simulink model "gm_DSBF"  (R2019b)
settings: Solver=FixedStepDiscrete  StartTime=0.0  StopTime=0.02  RelTol=1e-3
InitFcn:
  | sm_callback_init
StopFcn:
  | sm_callback_stop
undefined symbols (not defined in the file or in its folder): arraySize, arraySpacing, delayDataTypeFractionLength, delayDataTypeSign, delayDataTypeWordLength, mp, samplingRate, speedOfSound, upsampleFactor
libraries: hdlsllib x64, simulink x36, dspmlti4 x16, dsphdlfiltering x16
(part 3 of 5)

== system gm_DSBF/dataplane/Avalon Data Processing/delay signals_instance4/delay signal ==
  note: CIC interpolation
  note: Integer delay
  note: fractional delay (upsampled)
  data_in : Inport  OutDataTypeStr=fixdt(1, 32, 28)  PortDimensions=1  SampleTime=2.08333333333333e-05
  delay : Inport  Port=2  OutDataTypeStr=fixdt(1, 12, 6)  PortDimensions=1  SampleTime=2.08333333333333e-05
  CIC Interpolation : dspmlti4/CIC Interpolation  filtFrom=Filter object  filtobj=mp.cicInterpolator  ftype=Interpolator  R=mp.upsampleFactor  M=1  N=2  filterInternals=Full precision  BPS=[16 16 16 16]  FLPS=0  outputWordLength=32  outputFracLength=0  launchFVT=off  framing=Allow multirate processing  OutputFrames=off
      settings: SourceProductName=DSP System Toolbox  SourceProductBaseCode=DS
  CIC interpolation compensator : dsphdlfiltering/Discrete FIR Filter HDL Optimized  NumeratorSource=Property  Numerator=mp.cicInterpolatorCompensator.coeffs.Numerator  NumeratorPrototype=[]  FilterStructure=Direct form systolic  SerializationOption=Maximum number of multipliers  NumberOfCycles=2  NumberOfMultipliers=4  SimulateUsing=Code generation  roundingMode=Floor  overflowMode=off  CoefficientsDataTypeStr=fixdt(1,16)  CoefficientsMin=[]  CoefficientsMax=[]  OutputDataTypeStr=Inherit: Same word length as input  OutputMin=[]  OutputMax=[]  ResetInputPort=off  HDLGlobalReset=off
      settings: SourceProductName=DSP System Toolbox  SourceProductBaseCode=DS
  CIC interpolation gain compensation : ArithShift  BitShiftNumber=4  BinPtShiftNumber=double(0)
  Constant : Constant  OutDataTypeStr=boolean  SampleTime=-1
  Constant1 : Constant  OutDataTypeStr=boolean  SampleTime=-1
  Constant2 : Constant  OutDataTypeStr=boolean  SampleTime=-1
  Data Type Conversion : DataTypeConversion  OutDataTypeStr=fixdt(1, 32, 28)  SampleTime=1.30208333333333e-06
  Data Type Conversion1 : DataTypeConversion  OutDataTypeStr=fixdt(1, 32, 28)  SampleTime=2.08333333333333e-05
  Downsample : DownSample  N=double(16)  phase=double(0)  RateOptions=Allow multirate processing
  PipelineRegister : Delay  DelayLength=double(1)  InitialCondition=0  SampleTime=2.08333333333333e-05
  Rate Transition : RateTransition  InitialCondition=double(0)  OutPortSampleTimeOpt=Multiple of input port sample time  OutPortSampleTimeMultiple=1/16
  Rate Transition1 : RateTransition  InitialCondition=double(0)  OutPortSampleTimeOpt=Multiple of input port sample time  OutPortSampleTimeMultiple=1/2048
  Terminator2 : Terminator
  delayMatch{,1..3} (4 alike) : Delay  DelayLength=double(2)  InitialCondition=0  SampleTime=2.08333333333333e-05
  delayMatch4 : Delay  DelayLength=double(32)  InitialCondition=0  SampleTime=1.30208333333333e-06
  delayMatch5 : Delay  DelayLength=double(32)  InitialCondition=0  SampleTime=1.30208333333333e-06
  delayMatch6 : Delay  DelayLength=double(32)  InitialCondition=0  SampleTime=1.30208333333333e-06
  fractional delay DPRAM : hdlsllib/HDL RAMs/Simple Dual Port RAM  ram_size=mp.fractionalDelayAddrSize
      settings: SourceProductName=Simulink  SourceProductBaseCode=SL
  integer delay DPRAM : hdlsllib/HDL RAMs/Simple Dual Port RAM  ram_size=mp.integerDelayAddrSize
      settings: SourceProductName=Simulink  SourceProductBaseCode=SL
  read address generator : Subsystem
  read address generator1 : Subsystem
  split_into_int_and_frac_parts : Subsystem
  write address generator : hdlsllib/Sources/HDL Counter  CountType=Count limited  CountInit=double(0)  CountStep=double(1)  CountMax=double(63)  CountFromType=Initial value  CountFrom=double(0)  CountResetPort=off  CountLoadPort=off  CountEnbPort=off  CountDirPort=off  CountDataType=Unsigned  CountWordLen=6  CountFracLen=0  CountSampTime=2.08333333333333e-05
      settings: SourceProductName=Simulink
  write address generator1 : hdlsllib/Sources/HDL Counter  CountType=Count limited  CountInit=double(0)  CountStep=double(1)  CountMax=double(63)  CountFromType=Initial value  CountFrom=double(0)  CountResetPort=off  CountLoadPort=off  CountEnbPort=off  CountDirPort=off  CountDataType=Unsigned  CountWordLen=6  CountFracLen=0  CountSampTime=1.30208333333333e-06
      settings: SourceProductName=Simulink
  data_out : Outport  VectorParamsAs1DForOutWhenUnconnected=off
  wires:
  Downsample/1 -> PipelineRegister/1
  CIC interpolation gain compensation/1 -> Data Type Conversion/1
  split_into_int_and_frac_parts/1(integer_delay) -> read address generator/2(delay)
  Constant1/1 -> delayMatch6/1
  write address generator1/1 -> delayMatch4/1, delayMatch5/1
  delayMatch5/1 -> fractional delay DPRAM/2
  Constant/1 -> delayMatch3/1
  Constant2/1 -> delayMatch2/1
  write address generator/1 -> delayMatch/1, delayMatch1/1
  delayMatch1/1 -> integer delay DPRAM/2
  delay/1 -> split_into_int_and_frac_parts/1(delay)
  data_in/1 -> integer delay DPRAM/1
  delayMatch3/1 -> CIC interpolation compensator/2
  delayMatch6/1 -> fractional delay DPRAM/3
  delayMatch2/1 -> integer delay DPRAM/3
  Data Type Conversion/1 -> fractional delay DPRAM/1
  Data Type Conversion1/1 -> Rate Transition1/1
  split_into_int_and_frac_parts/2(fractional_delay) -> Rate Transition/1
  read address generator/1(read_addr) -> integer delay DPRAM/4
  read address generator1/1(read_addr) -> fractional delay DPRAM/4
  CIC Interpolation/1 -> CIC interpolation gain compensation/1
  CIC interpolation compensator/2 -> Terminator2/1
  CIC interpolation compensator/1 -> CIC Interpolation/1
  PipelineRegister/1 -> Data Type Conversion1/1
  Rate Transition/1 -> read address generator1/2(delay)
  Rate Transition1/1 -> data_out/1
  fractional delay DPRAM/1 -> Downsample/1
  integer delay DPRAM/1 -> CIC interpolation compensator/1
  delayMatch/1 -> read address generator/1(write_addr)
  delayMatch4/1 -> read address generator1/1(write_addr)

== system gm_DSBF/dataplane/Avalon Data Processing/delay signals_instance5/delay signal ==
  note: CIC interpolation
  note: Integer delay
  note: fractional delay (upsampled)
  data_in : Inport  OutDataTypeStr=fixdt(1, 32, 28)  PortDimensions=1  SampleTime=2.08333333333333e-05
  delay : Inport  Port=2  OutDataTypeStr=fixdt(1, 12, 6)  PortDimensions=1  SampleTime=2.08333333333333e-05
  CIC Interpolation : dspmlti4/CIC Interpolation  filtFrom=Filter object  filtobj=mp.cicInterpolator  ftype=Interpolator  R=mp.upsampleFactor  M=1  N=2  filterInternals=Full precision  BPS=[16 16 16 16]  FLPS=0  outputWordLength=32  outputFracLength=0  launchFVT=off  framing=Allow multirate processing  OutputFrames=off
      settings: SourceProductName=DSP System Toolbox  SourceProductBaseCode=DS
  CIC interpolation compensator : dsphdlfiltering/Discrete FIR Filter HDL Optimized  NumeratorSource=Property  Numerator=mp.cicInterpolatorCompensator.coeffs.Numerator  NumeratorPrototype=[]  FilterStructure=Direct form systolic  SerializationOption=Maximum number of multipliers  NumberOfCycles=2  NumberOfMultipliers=4  SimulateUsing=Code generation  roundingMode=Floor  overflowMode=off  CoefficientsDataTypeStr=fixdt(1,16)  CoefficientsMin=[]  CoefficientsMax=[]  OutputDataTypeStr=Inherit: Same word length as input  OutputMin=[]  OutputMax=[]  ResetInputPort=off  HDLGlobalReset=off
      settings: SourceProductName=DSP System Toolbox  SourceProductBaseCode=DS
  CIC interpolation gain compensation : ArithShift  BitShiftNumber=4  BinPtShiftNumber=double(0)
  Constant : Constant  OutDataTypeStr=boolean  SampleTime=-1
  Constant1 : Constant  OutDataTypeStr=boolean  SampleTime=-1
  Constant2 : Constant  OutDataTypeStr=boolean  SampleTime=-1
  Data Type Conversion : DataTypeConversion  OutDataTypeStr=fixdt(1, 32, 28)  SampleTime=1.30208333333333e-06
  Data Type Conversion1 : DataTypeConversion  OutDataTypeStr=fixdt(1, 32, 28)  SampleTime=2.08333333333333e-05
  Downsample : DownSample  N=double(16)  phase=double(0)  RateOptions=Allow multirate processing
  PipelineRegister : Delay  DelayLength=double(1)  InitialCondition=0  SampleTime=2.08333333333333e-05
  Rate Transition : RateTransition  InitialCondition=double(0)  OutPortSampleTimeOpt=Multiple of input port sample time  OutPortSampleTimeMultiple=1/16
  Rate Transition1 : RateTransition  InitialCondition=double(0)  OutPortSampleTimeOpt=Multiple of input port sample time  OutPortSampleTimeMultiple=1/2048
  Terminator2 : Terminator
  delayMatch{,1..3} (4 alike) : Delay  DelayLength=double(2)  InitialCondition=0  SampleTime=2.08333333333333e-05
  delayMatch4 : Delay  DelayLength=double(32)  InitialCondition=0  SampleTime=1.30208333333333e-06
  delayMatch5 : Delay  DelayLength=double(32)  InitialCondition=0  SampleTime=1.30208333333333e-06
  delayMatch6 : Delay  DelayLength=double(32)  InitialCondition=0  SampleTime=1.30208333333333e-06
  fractional delay DPRAM : hdlsllib/HDL RAMs/Simple Dual Port RAM  ram_size=mp.fractionalDelayAddrSize
      settings: SourceProductName=Simulink  SourceProductBaseCode=SL
  integer delay DPRAM : hdlsllib/HDL RAMs/Simple Dual Port RAM  ram_size=mp.integerDelayAddrSize
      settings: SourceProductName=Simulink  SourceProductBaseCode=SL
  read address generator : Subsystem
  read address generator1 : Subsystem
  split_into_int_and_frac_parts : Subsystem
  write address generator : hdlsllib/Sources/HDL Counter  CountType=Count limited  CountInit=double(0)  CountStep=double(1)  CountMax=double(63)  CountFromType=Initial value  CountFrom=double(0)  CountResetPort=off  CountLoadPort=off  CountEnbPort=off  CountDirPort=off  CountDataType=Unsigned  CountWordLen=6  CountFracLen=0  CountSampTime=2.08333333333333e-05
      settings: SourceProductName=Simulink
  write address generator1 : hdlsllib/Sources/HDL Counter  CountType=Count limited  CountInit=double(0)  CountStep=double(1)  CountMax=double(63)  CountFromType=Initial value  CountFrom=double(0)  CountResetPort=off  CountLoadPort=off  CountEnbPort=off  CountDirPort=off  CountDataType=Unsigned  CountWordLen=6  CountFracLen=0  CountSampTime=1.30208333333333e-06
      settings: SourceProductName=Simulink
  data_out : Outport  VectorParamsAs1DForOutWhenUnconnected=off
  wires:
  Downsample/1 -> PipelineRegister/1
  CIC interpolation gain compensation/1 -> Data Type Conversion/1
  split_into_int_and_frac_parts/1(integer_delay) -> read address generator/2(delay)
  Constant1/1 -> delayMatch6/1
  write address generator1/1 -> delayMatch4/1, delayMatch5/1
  delayMatch5/1 -> fractional delay DPRAM/2
  Constant/1 -> delayMatch3/1
  Constant2/1 -> delayMatch2/1
  write address generator/1 -> delayMatch/1, delayMatch1/1
  delayMatch1/1 -> integer delay DPRAM/2
  delay/1 -> split_into_int_and_frac_parts/1(delay)
  data_in/1 -> integer delay DPRAM/1
  delayMatch3/1 -> CIC interpolation compensator/2
  delayMatch6/1 -> fractional delay DPRAM/3
  delayMatch2/1 -> integer delay DPRAM/3
  Data Type Conversion/1 -> fractional delay DPRAM/1
  Data Type Conversion1/1 -> Rate Transition1/1
  split_into_int_and_frac_parts/2(fractional_delay) -> Rate Transition/1
  read address generator/1(read_addr) -> integer delay DPRAM/4
  read address generator1/1(read_addr) -> fractional delay DPRAM/4
  CIC Interpolation/1 -> CIC interpolation gain compensation/1
  CIC interpolation compensator/2 -> Terminator2/1
  CIC interpolation compensator/1 -> CIC Interpolation/1
  PipelineRegister/1 -> Data Type Conversion1/1
  Rate Transition/1 -> read address generator1/2(delay)
  Rate Transition1/1 -> data_out/1
  fractional delay DPRAM/1 -> Downsample/1
  integer delay DPRAM/1 -> CIC interpolation compensator/1
  delayMatch/1 -> read address generator/1(write_addr)
  delayMatch4/1 -> read address generator1/1(write_addr)

== system gm_DSBF/dataplane/Avalon Data Processing/delay signals_instance6/delay signal ==
  note: CIC interpolation
  note: Integer delay
  note: fractional delay (upsampled)
  data_in : Inport  OutDataTypeStr=fixdt(1, 32, 28)  PortDimensions=1  SampleTime=2.08333333333333e-05
  delay : Inport  Port=2  OutDataTypeStr=fixdt(1, 12, 6)  PortDimensions=1  SampleTime=2.08333333333333e-05
  CIC Interpolation : dspmlti4/CIC Interpolation  filtFrom=Filter object  filtobj=mp.cicInterpolator  ftype=Interpolator  R=mp.upsampleFactor  M=1  N=2  filterInternals=Full precision  BPS=[16 16 16 16]  FLPS=0  outputWordLength=32  outputFracLength=0  launchFVT=off  framing=Allow multirate processing  OutputFrames=off
      settings: SourceProductName=DSP System Toolbox  SourceProductBaseCode=DS
  CIC interpolation compensator : dsphdlfiltering/Discrete FIR Filter HDL Optimized  NumeratorSource=Property  Numerator=mp.cicInterpolatorCompensator.coeffs.Numerator  NumeratorPrototype=[]  FilterStructure=Direct form systolic  SerializationOption=Maximum number of multipliers  NumberOfCycles=2  NumberOfMultipliers=4  SimulateUsing=Code generation  roundingMode=Floor  overflowMode=off  CoefficientsDataTypeStr=fixdt(1,16)  CoefficientsMin=[]  CoefficientsMax=[]  OutputDataTypeStr=Inherit: Same word length as input  OutputMin=[]  OutputMax=[]  ResetInputPort=off  HDLGlobalReset=off
      settings: SourceProductName=DSP System Toolbox  SourceProductBaseCode=DS
  CIC interpolation gain compensation : ArithShift  BitShiftNumber=4  BinPtShiftNumber=double(0)
  Constant : Constant  OutDataTypeStr=boolean  SampleTime=-1
  Constant1 : Constant  OutDataTypeStr=boolean  SampleTime=-1
  Constant2 : Constant  OutDataTypeStr=boolean  SampleTime=-1
  Data Type Conversion : DataTypeConversion  OutDataTypeStr=fixdt(1, 32, 28)  SampleTime=1.30208333333333e-06
  Data Type Conversion1 : DataTypeConversion  OutDataTypeStr=fixdt(1, 32, 28)  SampleTime=2.08333333333333e-05
  Downsample : DownSample  N=double(16)  phase=double(0)  RateOptions=Allow multirate processing
  PipelineRegister : Delay  DelayLength=double(1)  InitialCondition=0  SampleTime=2.08333333333333e-05
  Rate Transition : RateTransition  InitialCondition=double(0)  OutPortSampleTimeOpt=Multiple of input port sample time  OutPortSampleTimeMultiple=1/16
  Rate Transition1 : RateTransition  InitialCondition=double(0)  OutPortSampleTimeOpt=Multiple of input port sample time  OutPortSampleTimeMultiple=1/2048
  Terminator2 : Terminator
  delayMatch{,1..3} (4 alike) : Delay  DelayLength=double(2)  InitialCondition=0  SampleTime=2.08333333333333e-05
  delayMatch4 : Delay  DelayLength=double(32)  InitialCondition=0  SampleTime=1.30208333333333e-06
  delayMatch5 : Delay  DelayLength=double(32)  InitialCondition=0  SampleTime=1.30208333333333e-06
  delayMatch6 : Delay  DelayLength=double(32)  InitialCondition=0  SampleTime=1.30208333333333e-06
  fractional delay DPRAM : hdlsllib/HDL RAMs/Simple Dual Port RAM  ram_size=mp.fractionalDelayAddrSize
      settings: SourceProductName=Simulink  SourceProductBaseCode=SL
  integer delay DPRAM : hdlsllib/HDL RAMs/Simple Dual Port RAM  ram_size=mp.integerDelayAddrSize
      settings: SourceProductName=Simulink  SourceProductBaseCode=SL
  read address generator : Subsystem
  read address generator1 : Subsystem
  split_into_int_and_frac_parts : Subsystem
  write address generator : hdlsllib/Sources/HDL Counter  CountType=Count limited  CountInit=double(0)  CountStep=double(1)  CountMax=double(63)  CountFromType=Initial value  CountFrom=double(0)  CountResetPort=off  CountLoadPort=off  CountEnbPort=off  CountDirPort=off  CountDataType=Unsigned  CountWordLen=6  CountFracLen=0  CountSampTime=2.08333333333333e-05
      settings: SourceProductName=Simulink
  write address generator1 : hdlsllib/Sources/HDL Counter  CountType=Count limited  CountInit=double(0)  CountStep=double(1)  CountMax=double(63)  CountFromType=Initial value  CountFrom=double(0)  CountResetPort=off  CountLoadPort=off  CountEnbPort=off  CountDirPort=off  CountDataType=Unsigned  CountWordLen=6  CountFracLen=0  CountSampTime=1.30208333333333e-06
      settings: SourceProductName=Simulink
  data_out : Outport  VectorParamsAs1DForOutWhenUnconnected=off
  wires:
  Downsample/1 -> PipelineRegister/1
  CIC interpolation gain compensation/1 -> Data Type Conversion/1
  split_into_int_and_frac_parts/1(integer_delay) -> read address generator/2(delay)
  Constant1/1 -> delayMatch6/1
  write address generator1/1 -> delayMatch4/1, delayMatch5/1
  delayMatch5/1 -> fractional delay DPRAM/2
  Constant/1 -> delayMatch3/1
  Constant2/1 -> delayMatch2/1
  write address generator/1 -> delayMatch/1, delayMatch1/1
  delayMatch1/1 -> integer delay DPRAM/2
  delay/1 -> split_into_int_and_frac_parts/1(delay)
  data_in/1 -> integer delay DPRAM/1
  delayMatch3/1 -> CIC interpolation compensator/2
  delayMatch6/1 -> fractional delay DPRAM/3
  delayMatch2/1 -> integer delay DPRAM/3
  Data Type Conversion/1 -> fractional delay DPRAM/1
  Data Type Conversion1/1 -> Rate Transition1/1
  split_into_int_and_frac_parts/2(fractional_delay) -> Rate Transition/1
  read address generator/1(read_addr) -> integer delay DPRAM/4
  read address generator1/1(read_addr) -> fractional delay DPRAM/4
  CIC Interpolation/1 -> CIC interpolation gain compensation/1
  CIC interpolation compensator/2 -> Terminator2/1
  CIC interpolation compensator/1 -> CIC Interpolation/1
  PipelineRegister/1 -> Data Type Conversion1/1
  Rate Transition/1 -> read address generator1/2(delay)
  Rate Transition1/1 -> data_out/1
  fractional delay DPRAM/1 -> Downsample/1
  integer delay DPRAM/1 -> CIC interpolation compensator/1
  delayMatch/1 -> read address generator/1(write_addr)
  delayMatch4/1 -> read address generator1/1(write_addr)

== system gm_DSBF/dataplane/Avalon Data Processing/delay signals_instance7/delay signal ==
  note: CIC interpolation
  note: Integer delay
  note: fractional delay (upsampled)
  data_in : Inport  OutDataTypeStr=fixdt(1, 32, 28)  PortDimensions=1  SampleTime=2.08333333333333e-05
  delay : Inport  Port=2  OutDataTypeStr=fixdt(1, 12, 6)  PortDimensions=1  SampleTime=2.08333333333333e-05
  CIC Interpolation : dspmlti4/CIC Interpolation  filtFrom=Filter object  filtobj=mp.cicInterpolator  ftype=Interpolator  R=mp.upsampleFactor  M=1  N=2  filterInternals=Full precision  BPS=[16 16 16 16]  FLPS=0  outputWordLength=32  outputFracLength=0  launchFVT=off  framing=Allow multirate processing  OutputFrames=off
      settings: SourceProductName=DSP System Toolbox  SourceProductBaseCode=DS
  CIC interpolation compensator : dsphdlfiltering/Discrete FIR Filter HDL Optimized  NumeratorSource=Property  Numerator=mp.cicInterpolatorCompensator.coeffs.Numerator  NumeratorPrototype=[]  FilterStructure=Direct form systolic  SerializationOption=Maximum number of multipliers  NumberOfCycles=2  NumberOfMultipliers=4  SimulateUsing=Code generation  roundingMode=Floor  overflowMode=off  CoefficientsDataTypeStr=fixdt(1,16)  CoefficientsMin=[]  CoefficientsMax=[]  OutputDataTypeStr=Inherit: Same word length as input  OutputMin=[]  OutputMax=[]  ResetInputPort=off  HDLGlobalReset=off
      settings: SourceProductName=DSP System Toolbox  SourceProductBaseCode=DS
  CIC interpolation gain compensation : ArithShift  BitShiftNumber=4  BinPtShiftNumber=double(0)
  Constant : Constant  OutDataTypeStr=boolean  SampleTime=-1
  Constant1 : Constant  OutDataTypeStr=boolean  SampleTime=-1
  Constant2 : Constant  OutDataTypeStr=boolean  SampleTime=-1
  Data Type Conversion : DataTypeConversion  OutDataTypeStr=fixdt(1, 32, 28)  SampleTime=1.30208333333333e-06
  Data Type Conversion1 : DataTypeConversion  OutDataTypeStr=fixdt(1, 32, 28)  SampleTime=2.08333333333333e-05
  Downsample : DownSample  N=double(16)  phase=double(0)  RateOptions=Allow multirate processing
  PipelineRegister : Delay  DelayLength=double(1)  InitialCondition=0  SampleTime=2.08333333333333e-05
  Rate Transition : RateTransition  InitialCondition=double(0)  OutPortSampleTimeOpt=Multiple of input port sample time  OutPortSampleTimeMultiple=1/16
  Rate Transition1 : RateTransition  InitialCondition=double(0)  OutPortSampleTimeOpt=Multiple of input port sample time  OutPortSampleTimeMultiple=1/2048
  Terminator2 : Terminator
  delayMatch{,1..3} (4 alike) : Delay  DelayLength=double(2)  InitialCondition=0  SampleTime=2.08333333333333e-05
  delayMatch4 : Delay  DelayLength=double(32)  InitialCondition=0  SampleTime=1.30208333333333e-06
  delayMatch5 : Delay  DelayLength=double(32)  InitialCondition=0  SampleTime=1.30208333333333e-06
  delayMatch6 : Delay  DelayLength=double(32)  InitialCondition=0  SampleTime=1.30208333333333e-06
  fractional delay DPRAM : hdlsllib/HDL RAMs/Simple Dual Port RAM  ram_size=mp.fractionalDelayAddrSize
      settings: SourceProductName=Simulink  SourceProductBaseCode=SL
  integer delay DPRAM : hdlsllib/HDL RAMs/Simple Dual Port RAM  ram_size=mp.integerDelayAddrSize
      settings: SourceProductName=Simulink  SourceProductBaseCode=SL
  read address generator : Subsystem
  read address generator1 : Subsystem
  split_into_int_and_frac_parts : Subsystem
  write address generator : hdlsllib/Sources/HDL Counter  CountType=Count limited  CountInit=double(0)  CountStep=double(1)  CountMax=double(63)  CountFromType=Initial value  CountFrom=double(0)  CountResetPort=off  CountLoadPort=off  CountEnbPort=off  CountDirPort=off  CountDataType=Unsigned  CountWordLen=6  CountFracLen=0  CountSampTime=2.08333333333333e-05
      settings: SourceProductName=Simulink
  write address generator1 : hdlsllib/Sources/HDL Counter  CountType=Count limited  CountInit=double(0)  CountStep=double(1)  CountMax=double(63)  CountFromType=Initial value  CountFrom=double(0)  CountResetPort=off  CountLoadPort=off  CountEnbPort=off  CountDirPort=off  CountDataType=Unsigned  CountWordLen=6  CountFracLen=0  CountSampTime=1.30208333333333e-06
      settings: SourceProductName=Simulink
  data_out : Outport  VectorParamsAs1DForOutWhenUnconnected=off
  wires:
  Downsample/1 -> PipelineRegister/1
  CIC interpolation gain compensation/1 -> Data Type Conversion/1
  split_into_int_and_frac_parts/1(integer_delay) -> read address generator/2(delay)
  Constant1/1 -> delayMatch6/1
  write address generator1/1 -> delayMatch4/1, delayMatch5/1
  delayMatch5/1 -> fractional delay DPRAM/2
  Constant/1 -> delayMatch3/1
  Constant2/1 -> delayMatch2/1
  write address generator/1 -> delayMatch/1, delayMatch1/1
  delayMatch1/1 -> integer delay DPRAM/2
  delay/1 -> split_into_int_and_frac_parts/1(delay)
  data_in/1 -> integer delay DPRAM/1
  delayMatch3/1 -> CIC interpolation compensator/2
  delayMatch6/1 -> fractional delay DPRAM/3
  delayMatch2/1 -> integer delay DPRAM/3
  Data Type Conversion/1 -> fractional delay DPRAM/1
  Data Type Conversion1/1 -> Rate Transition1/1
  split_into_int_and_frac_parts/2(fractional_delay) -> Rate Transition/1
  read address generator/1(read_addr) -> integer delay DPRAM/4
  read address generator1/1(read_addr) -> fractional delay DPRAM/4
  CIC Interpolation/1 -> CIC interpolation gain compensation/1
  CIC interpolation compensator/2 -> Terminator2/1
  CIC interpolation compensator/1 -> CIC Interpolation/1
  PipelineRegister/1 -> Data Type Conversion1/1
  Rate Transition/1 -> read address generator1/2(delay)
  Rate Transition1/1 -> data_out/1
  fractional delay DPRAM/1 -> Downsample/1
  integer delay DPRAM/1 -> CIC interpolation compensator/1
  delayMatch/1 -> read address generator/1(write_addr)
  delayMatch4/1 -> read address generator1/1(write_addr)

== system gm_DSBF/dataplane/Avalon Data Processing/delay signals_instance8/delay signal ==
  note: CIC interpolation
  note: Integer delay
  note: fractional delay (upsampled)
  data_in : Inport  OutDataTypeStr=fixdt(1, 32, 28)  PortDimensions=1  SampleTime=2.08333333333333e-05
  delay : Inport  Port=2  OutDataTypeStr=fixdt(1, 12, 6)  PortDimensions=1  SampleTime=2.08333333333333e-05
  CIC Interpolation : dspmlti4/CIC Interpolation  filtFrom=Filter object  filtobj=mp.cicInterpolator  ftype=Interpolator  R=mp.upsampleFactor  M=1  N=2  filterInternals=Full precision  BPS=[16 16 16 16]  FLPS=0  outputWordLength=32  outputFracLength=0  launchFVT=off  framing=Allow multirate processing  OutputFrames=off
      settings: SourceProductName=DSP System Toolbox  SourceProductBaseCode=DS
  CIC interpolation compensator : dsphdlfiltering/Discrete FIR Filter HDL Optimized  NumeratorSource=Property  Numerator=mp.cicInterpolatorCompensator.coeffs.Numerator  NumeratorPrototype=[]  FilterStructure=Direct form systolic  SerializationOption=Maximum number of multipliers  NumberOfCycles=2  NumberOfMultipliers=4  SimulateUsing=Code generation  roundingMode=Floor  overflowMode=off  CoefficientsDataTypeStr=fixdt(1,16)  CoefficientsMin=[]  CoefficientsMax=[]  OutputDataTypeStr=Inherit: Same word length as input  OutputMin=[]  OutputMax=[]  ResetInputPort=off  HDLGlobalReset=off
      settings: SourceProductName=DSP System Toolbox  SourceProductBaseCode=DS
  CIC interpolation gain compensation : ArithShift  BitShiftNumber=4  BinPtShiftNumber=double(0)
  Constant : Constant  OutDataTypeStr=boolean  SampleTime=-1
  Constant1 : Constant  OutDataTypeStr=boolean  SampleTime=-1
  Constant2 : Constant  OutDataTypeStr=boolean  SampleTime=-1
  Data Type Conversion : DataTypeConversion  OutDataTypeStr=fixdt(1, 32, 28)  SampleTime=1.30208333333333e-06
  Data Type Conversion1 : DataTypeConversion  OutDataTypeStr=fixdt(1, 32, 28)  SampleTime=2.08333333333333e-05
  Downsample : DownSample  N=double(16)  phase=double(0)  RateOptions=Allow multirate processing
  PipelineRegister : Delay  DelayLength=double(1)  InitialCondition=0  SampleTime=2.08333333333333e-05
  Rate Transition : RateTransition  InitialCondition=double(0)  OutPortSampleTimeOpt=Multiple of input port sample time  OutPortSampleTimeMultiple=1/16
  Rate Transition1 : RateTransition  InitialCondition=double(0)  OutPortSampleTimeOpt=Multiple of input port sample time  OutPortSampleTimeMultiple=1/2048
  Terminator2 : Terminator
  delayMatch{,1..3} (4 alike) : Delay  DelayLength=double(2)  InitialCondition=0  SampleTime=2.08333333333333e-05
  delayMatch4 : Delay  DelayLength=double(32)  InitialCondition=0  SampleTime=1.30208333333333e-06
  delayMatch5 : Delay  DelayLength=double(32)  InitialCondition=0  SampleTime=1.30208333333333e-06
  delayMatch6 : Delay  DelayLength=double(32)  InitialCondition=0  SampleTime=1.30208333333333e-06
  fractional delay DPRAM : hdlsllib/HDL RAMs/Simple Dual Port RAM  ram_size=mp.fractionalDelayAddrSize
      settings: SourceProductName=Simulink  SourceProductBaseCode=SL
  integer delay DPRAM : hdlsllib/HDL RAMs/Simple Dual Port RAM  ram_size=mp.integerDelayAddrSize
      settings: SourceProductName=Simulink  SourceProductBaseCode=SL
  read address generator : Subsystem
  read address generator1 : Subsystem
  split_into_int_and_frac_parts : Subsystem
  write address generator : hdlsllib/Sources/HDL Counter  CountType=Count limited  CountInit=double(0)  CountStep=double(1)  CountMax=double(63)  CountFromType=Initial value  CountFrom=double(0)  CountResetPort=off  CountLoadPort=off  CountEnbPort=off  CountDirPort=off  CountDataType=Unsigned  CountWordLen=6  CountFracLen=0  CountSampTime=2.08333333333333e-05
      settings: SourceProductName=Simulink
  write address generator1 : hdlsllib/Sources/HDL Counter  CountType=Count limited  CountInit=double(0)  CountStep=double(1)  CountMax=double(63)  CountFromType=Initial value  CountFrom=double(0)  CountResetPort=off  CountLoadPort=off  CountEnbPort=off  CountDirPort=off  CountDataType=Unsigned  CountWordLen=6  CountFracLen=0  CountSampTime=1.30208333333333e-06
      settings: SourceProductName=Simulink
  data_out : Outport  VectorParamsAs1DForOutWhenUnconnected=off
  wires:
  Downsample/1 -> PipelineRegister/1
  CIC interpolation gain compensation/1 -> Data Type Conversion/1
  split_into_int_and_frac_parts/1(integer_delay) -> read address generator/2(delay)
  Constant1/1 -> delayMatch6/1
  write address generator1/1 -> delayMatch4/1, delayMatch5/1
  delayMatch5/1 -> fractional delay DPRAM/2
  Constant/1 -> delayMatch3/1
  Constant2/1 -> delayMatch2/1
  write address generator/1 -> delayMatch/1, delayMatch1/1
  delayMatch1/1 -> integer delay DPRAM/2
  delay/1 -> split_into_int_and_frac_parts/1(delay)
  data_in/1 -> integer delay DPRAM/1
  delayMatch3/1 -> CIC interpolation compensator/2
  delayMatch6/1 -> fractional delay DPRAM/3
  delayMatch2/1 -> integer delay DPRAM/3
  Data Type Conversion/1 -> fractional delay DPRAM/1
  Data Type Conversion1/1 -> Rate Transition1/1
  split_into_int_and_frac_parts/2(fractional_delay) -> Rate Transition/1
  read address generator/1(read_addr) -> integer delay DPRAM/4
  read address generator1/1(read_addr) -> fractional delay DPRAM/4
  CIC Interpolation/1 -> CIC interpolation gain compensation/1
  CIC interpolation compensator/2 -> Terminator2/1
  CIC interpolation compensator/1 -> CIC Interpolation/1
  PipelineRegister/1 -> Data Type Conversion1/1
  Rate Transition/1 -> read address generator1/2(delay)
  Rate Transition1/1 -> data_out/1
  fractional delay DPRAM/1 -> Downsample/1
  integer delay DPRAM/1 -> CIC interpolation compensator/1
  delayMatch/1 -> read address generator/1(write_addr)
  delayMatch4/1 -> read address generator1/1(write_addr)

== system gm_DSBF/dataplane/Avalon Data Processing/delay signals_instance9/delay signal ==
  note: CIC interpolation
  note: Integer delay
  note: fractional delay (upsampled)
  data_in : Inport  OutDataTypeStr=fixdt(1, 32, 28)  PortDimensions=1  SampleTime=2.08333333333333e-05
  delay : Inport  Port=2  OutDataTypeStr=fixdt(1, 12, 6)  PortDimensions=1  SampleTime=2.08333333333333e-05
  CIC Interpolation : dspmlti4/CIC Interpolation  filtFrom=Filter object  filtobj=mp.cicInterpolator  ftype=Interpolator  R=mp.upsampleFactor  M=1  N=2  filterInternals=Full precision  BPS=[16 16 16 16]  FLPS=0  outputWordLength=32  outputFracLength=0  launchFVT=off  framing=Allow multirate processing  OutputFrames=off
      settings: SourceProductName=DSP System Toolbox  SourceProductBaseCode=DS
  CIC interpolation compensator : dsphdlfiltering/Discrete FIR Filter HDL Optimized  NumeratorSource=Property  Numerator=mp.cicInterpolatorCompensator.coeffs.Numerator  NumeratorPrototype=[]  FilterStructure=Direct form systolic  SerializationOption=Maximum number of multipliers  NumberOfCycles=2  NumberOfMultipliers=4  SimulateUsing=Code generation  roundingMode=Floor  overflowMode=off  CoefficientsDataTypeStr=fixdt(1,16)  CoefficientsMin=[]  CoefficientsMax=[]  OutputDataTypeStr=Inherit: Same word length as input  OutputMin=[]  OutputMax=[]  ResetInputPort=off  HDLGlobalReset=off
      settings: SourceProductName=DSP System Toolbox  SourceProductBaseCode=DS
  CIC interpolation gain compensation : ArithShift  BitShiftNumber=4  BinPtShiftNumber=double(0)
  Constant : Constant  OutDataTypeStr=boolean  SampleTime=-1
  Constant1 : Constant  OutDataTypeStr=boolean  SampleTime=-1
  Constant2 : Constant  OutDataTypeStr=boolean  SampleTime=-1
  Data Type Conversion : DataTypeConversion  OutDataTypeStr=fixdt(1, 32, 28)  SampleTime=1.30208333333333e-06
  Data Type Conversion1 : DataTypeConversion  OutDataTypeStr=fixdt(1, 32, 28)  SampleTime=2.08333333333333e-05
  Downsample : DownSample  N=double(16)  phase=double(0)  RateOptions=Allow multirate processing
  PipelineRegister : Delay  DelayLength=double(1)  InitialCondition=0  SampleTime=2.08333333333333e-05
  Rate Transition : RateTransition  InitialCondition=double(0)  OutPortSampleTimeOpt=Multiple of input port sample time  OutPortSampleTimeMultiple=1/16
  Rate Transition1 : RateTransition  InitialCondition=double(0)  OutPortSampleTimeOpt=Multiple of input port sample time  OutPortSampleTimeMultiple=1/2048
  Terminator2 : Terminator
  delayMatch{,1..3} (4 alike) : Delay  DelayLength=double(2)  InitialCondition=0  SampleTime=2.08333333333333e-05
  delayMatch4 : Delay  DelayLength=double(32)  InitialCondition=0  SampleTime=1.30208333333333e-06
  delayMatch5 : Delay  DelayLength=double(32)  InitialCondition=0  SampleTime=1.30208333333333e-06
  delayMatch6 : Delay  DelayLength=double(32)  InitialCondition=0  SampleTime=1.30208333333333e-06
  fractional delay DPRAM : hdlsllib/HDL RAMs/Simple Dual Port RAM  ram_size=mp.fractionalDelayAddrSize
      settings: SourceProductName=Simulink  SourceProductBaseCode=SL
  integer delay DPRAM : hdlsllib/HDL RAMs/Simple Dual Port RAM  ram_size=mp.integerDelayAddrSize
      settings: SourceProductName=Simulink  SourceProductBaseCode=SL
  read address generator : Subsystem
  read address generator1 : Subsystem
  split_into_int_and_frac_parts : Subsystem
  write address generator : hdlsllib/Sources/HDL Counter  CountType=Count limited  CountInit=double(0)  CountStep=double(1)  CountMax=double(63)  CountFromType=Initial value  CountFrom=double(0)  CountResetPort=off  CountLoadPort=off  CountEnbPort=off  CountDirPort=off  CountDataType=Unsigned  CountWordLen=6  CountFracLen=0  CountSampTime=2.08333333333333e-05
      settings: SourceProductName=Simulink
  write address generator1 : hdlsllib/Sources/HDL Counter  CountType=Count limited  CountInit=double(0)  CountStep=double(1)  CountMax=double(63)  CountFromType=Initial value  CountFrom=double(0)  CountResetPort=off  CountLoadPort=off  CountEnbPort=off  CountDirPort=off  CountDataType=Unsigned  CountWordLen=6  CountFracLen=0  CountSampTime=1.30208333333333e-06
      settings: SourceProductName=Simulink
  data_out : Outport  VectorParamsAs1DForOutWhenUnconnected=off
  wires:
  Downsample/1 -> PipelineRegister/1
  CIC interpolation gain compensation/1 -> Data Type Conversion/1
  split_into_int_and_frac_parts/1(integer_delay) -> read address generator/2(delay)
  Constant1/1 -> delayMatch6/1
  write address generator1/1 -> delayMatch4/1, delayMatch5/1
  delayMatch5/1 -> fractional delay DPRAM/2
  Constant/1 -> delayMatch3/1
  Constant2/1 -> delayMatch2/1
  write address generator/1 -> delayMatch/1, delayMatch1/1
  delayMatch1/1 -> integer delay DPRAM/2
  delay/1 -> split_into_int_and_frac_parts/1(delay)
  data_in/1 -> integer delay DPRAM/1
  delayMatch3/1 -> CIC interpolation compensator/2
  delayMatch6/1 -> fractional delay DPRAM/3
  delayMatch2/1 -> integer delay DPRAM/3
  Data Type Conversion/1 -> fractional delay DPRAM/1
  Data Type Conversion1/1 -> Rate Transition1/1
  split_into_int_and_frac_parts/2(fractional_delay) -> Rate Transition/1
  read address generator/1(read_addr) -> integer delay DPRAM/4
  read address generator1/1(read_addr) -> fractional delay DPRAM/4
  CIC Interpolation/1 -> CIC interpolation gain compensation/1
  CIC interpolation compensator/2 -> Terminator2/1
  CIC interpolation compensator/1 -> CIC Interpolation/1
  PipelineRegister/1 -> Data Type Conversion1/1
  Rate Transition/1 -> read address generator1/2(delay)
  Rate Transition1/1 -> data_out/1
  fractional delay DPRAM/1 -> Downsample/1
  integer delay DPRAM/1 -> CIC interpolation compensator/1
  delayMatch/1 -> read address generator/1(write_addr)
  delayMatch4/1 -> read address generator1/1(write_addr)

== system gm_DSBF/dataplane/Avalon Data Processing/normalize/normalize_shift ==
  input : Inport  OutDataTypeStr=fixdt(1, 36, 28)  PortDimensions=1  SampleTime=1.01725260416667e-08
  normalize_shift : MATLAB Function  TreatAsAtomicUnit=on
  normalized : Outport  VectorParamsAs1DForOutWhenUnconnected=off
  wires:
  normalize_shift/1(normalized) -> normalized/1
  input/1 -> normalize_shift/1(input)

== system gm_DSBF/dataplane/compute projections/compute cosine/cos LUT ==
  In1 : Inport  OutDataTypeStr=fixdt(1, 16, 8)  PortDimensions=1  SampleTime=1.01725260416667e-08
  DTC1 : DataTypeConversion  RndMeth=Nearest
  LUT : Lookup_n-D  NumberOfTableDimensions=1  LookupTableObject=FunctionApproximation_LUTObject_20200313T090826873  BreakpointsSpecification=Even spacing  BreakpointsForDimension3=[5, 7]  BreakpointsForDimension1FirstPoint=0  BreakpointsForDimension1Spacing=2  IndexSearchMethod=Evenly spaced points  Table=[1 0.9993896484375 0.99755859375 0.9945068359375 0.99029541015625 0.98480224609375 0.9781494140625 0.97027587890625 0.96124267578125 0.9510498046875 0.939697265625 0.92718505859375 0.91357421875 0.8988037109375 0.8829345703125 0.86602783203125 0.8480224609375 0.82904052734375 0.80902099609375 0.78802490234375 0.76605224609375 0.7431640625 0.7193603515625 0.69464111328125 0.66912841796875 0.64276123046875 0.61566162109375 0.5877685546875 0.5592041015625 0.5299072265625 0.5 0.469482421875 0.4383544921875 0.40673828125 0.3746337890625 0.342041015625 0.30902099609375 0.275634765625 0.241943359375 0.2078857421875 0.17364501953125 0.13916015625 0.10455322265625 0.06976318359375 0.034912109375 0]  TableDataTypeStr=numerictype(1,16,14)  ExtrapMethod=Clip  DiagnosticForOutOfRangeInput=Error  UseLastTableValue=on  InternalRulePriority=Speed  OutDataTypeStr=numerictype(1,16,14)  RndMeth=Simplest
  SigSpec1 : SignalSpecification  OutMin=0  OutMax=90  OutDataTypeStr=numerictype(1,16,8)
  Out1 : Outport
  wires:
  DTC1/1 -> SigSpec1/1
  LUT/1 -> Out1/1
  SigSpec1/1 -> LUT/1
  In1/1 -> DTC1/1

== system gm_DSBF/dataplane/compute projections/compute sine/sin LUT ==
  angle : Inport  OutDataTypeStr=fixdt(1, 16, 8)  PortDimensions=1  SampleTime=1.01725260416667e-08
  DTC2 : DataTypeConversion  RndMeth=Nearest
  LUT1 : Lookup_n-D  NumberOfTableDimensions=1  LookupTableObject=FunctionApproximation_LUTObject_20200313T084211896  BreakpointsSpecification=Even spacing  BreakpointsForDimension3=[5, 7]  BreakpointsForDimension1FirstPoint=0  BreakpointsForDimension1Spacing=4  IndexSearchMethod=Evenly spaced points  Table=[0 0.06976318359375 0.13916015625 0.2078857421875 0.275634765625 0.342041015625 0.40673828125 0.469482421875 0.5299072265625 0.5877685546875 0.64276123046875 0.69464111328125 0.7431640625 0.78802490234375 0.82904052734375 0.86602783203125 0.8988037109375 0.92718505859375 0.9510498046875 0.97027587890625 0.98480224609375 0.9945068359375 0.9993896484375]  TableDataTypeStr=numerictype(1,16,14)  ExtrapMethod=Clip  DiagnosticForOutOfRangeInput=Error  UseLastTableValue=on  InternalRulePriority=Speed  OutDataTypeStr=numerictype(1,16,14)  RndMeth=Simplest
  SigSpec2 : SignalSpecification  OutMin=0  OutMax=90  OutDataTypeStr=numerictype(1,16,8)
  sin_angle : Outport
  wires:
  DTC2/1 -> SigSpec2/1
  LUT1/1 -> sin_angle/1
  SigSpec2/1 -> LUT1/1
  angle/1 -> DTC2/1

== system gm_DSBF/dataplane/compute projections/compute sine1/sin LUT ==
  angle : Inport  OutDataTypeStr=fixdt(1, 16, 8)  PortDimensions=1  SampleTime=1.01725260416667e-08
  DTC2 : DataTypeConversion  RndMeth=Nearest
  LUT1 : Lookup_n-D  NumberOfTableDimensions=1  LookupTableObject=FunctionApproximation_LUTObject_20200313T084211896  BreakpointsSpecification=Even spacing  BreakpointsForDimension3=[5, 7]  BreakpointsForDimension1FirstPoint=0  BreakpointsForDimension1Spacing=4  IndexSearchMethod=Evenly spaced points  Table=[0 0.06976318359375 0.13916015625 0.2078857421875 0.275634765625 0.342041015625 0.40673828125 0.469482421875 0.5299072265625 0.5877685546875 0.64276123046875 0.69464111328125 0.7431640625 0.78802490234375 0.82904052734375 0.86602783203125 0.8988037109375 0.92718505859375 0.9510498046875 0.97027587890625 0.98480224609375 0.9945068359375 0.9993896484375]  TableDataTypeStr=numerictype(1,16,14)  ExtrapMethod=Clip  DiagnosticForOutOfRangeInput=Error  UseLastTableValue=on  InternalRulePriority=Speed  OutDataTypeStr=numerictype(1,16,14)  RndMeth=Simplest
  SigSpec2 : SignalSpecification  OutMin=0  OutMax=90  OutDataTypeStr=numerictype(1,16,8)
  sin_angle : Outport
  wires:
  DTC2/1 -> SigSpec2/1
  LUT1/1 -> sin_angle/1
  SigSpec2/1 -> LUT1/1
  angle/1 -> DTC2/1

== system gm_DSBF/dataplane/Avalon Data Processing/delay signals_instance1/delay signal/read address generator ==
  note: wrap on overflow is the desired behavior
  note: this offset is the maximum possible delay from a microphone to the the center of the array
  note: To accommodate positive and negative delays, the read pointer needs to lag the write pointer by the maximum delay + 1. For the maximum positive delay, this puts the read pointer 1 behind the write pointer.
  write_addr : Inport  OutDataTypeStr=fixdt(0, 6, 0)  PortDimensions=1  SampleTime=2.08333333333333e-05
  delay : Inport  Port=2  OutDataTypeStr=fixdt(1, 6, 0)  PortDimensions=1  SampleTime=2.08333333333333e-05
  Increment Real World : simulink/Additional Math & Discrete/Additional Math: Increment - Decrement/Increment Real World
      settings: SourceProductName=Simulink  SourceProductBaseCode=SL
  Subtract : Subsystem
  phase center reference offset : Constant  Value=fix(mp.maxDelay/2)  OutDataTypeStr=fixdt(0,delayDataTypeWordLength - delayDataTypeFractionLength,0)  SampleTime=-1
  read_addr : Outport  VectorParamsAs1DForOutWhenUnconnected=off
  wires:
  phase center reference offset/1 -> Increment Real World/1
  Subtract/1(Out1) -> read_addr/1
  Increment Real World/1 -> Subtract/3(In3)
  write_addr/1 -> Subtract/2(In2)
  delay/1 -> Subtract/1(In1)

== system gm_DSBF/dataplane/Avalon Data Processing/delay signals_instance1/delay signal/read address generator1 ==
  note: this offset is the maximum possible delay from a microphone to the the center of the array
  note: To accommodate positive and negative delays, the read pointer needs to lag the write pointer by the maximum delay + 1. For the maximum positive delay, this puts the read pointer 1 behind the write pointer.
  note: wrap on overflow is the desired behavior
  write_addr : Inport  OutDataTypeStr=fixdt(0, 6, 0)  PortDimensions=1  SampleTime=1.30208333333333e-06
  delay : Inport  Port=2  OutDataTypeStr=fixdt(1, 6, 0)  PortDimensions=1  SampleTime=1.30208333333333e-06
  Increment Real World : simulink/Additional Math & Discrete/Additional Math: Increment - Decrement/Increment Real World
      settings: SourceProductName=Simulink  SourceProductBaseCode=SL
  Subtract : Subsystem
  phase center reference offset : Constant  Value=fix(mp.upsampleFactor)  OutDataTypeStr=fixdt(0, delayDataTypeFractionLength, 0)  SampleTime=-1
  read_addr : Outport  VectorParamsAs1DForOutWhenUnconnected=off
  wires:
  phase center reference offset/1 -> Increment Real World/1
  Subtract/1(Out1) -> read_addr/1
  Increment Real World/1 -> Subtract/3(In3)
  write_addr/1 -> Subtract/2(In2)
  delay/1 -> Subtract/1(In1)

== system gm_DSBF/dataplane/Avalon Data Processing/delay signals_instance1/delay signal/split_into_int_and_frac_parts ==
  delay : Inport  OutDataTypeStr=fixdt(1, 12, 6)  PortDimensions=1  SampleTime=2.08333333333333e-05
  split_into_int_and_frac_parts : MATLAB Function  TreatAsAtomicUnit=on
  integer_delay : Outport  VectorParamsAs1DForOutWhenUnconnected=off
  fractional_delay : Outport  Port=2
  wires:
  split_into_int_and_frac_parts/1(integer_delay) -> integer_delay/1
  split_into_int_and_frac_parts/2(fractional_delay) -> fractional_delay/1
  delay/1 -> split_into_int_and_frac_parts/1(delay)

== system gm_DSBF/dataplane/Avalon Data Processing/delay signals_instance10/delay signal/read address generator ==
  note: To accommodate positive and negative delays, the read pointer needs to lag the write pointer by the maximum delay + 1. For the maximum positive delay, this puts the read pointer 1 behind the write pointer.
  note: this offset is the maximum possible delay from a microphone to the the center of the array
  note: wrap on overflow is the desired behavior
  write_addr : Inport  OutDataTypeStr=fixdt(0, 6, 0)  PortDimensions=1  SampleTime=2.08333333333333e-05
  delay : Inport  Port=2  OutDataTypeStr=fixdt(1, 6, 0)  PortDimensions=1  SampleTime=2.08333333333333e-05
  Increment Real World : simulink/Additional Math & Discrete/Additional Math: Increment - Decrement/Increment Real World
      settings: SourceProductName=Simulink  SourceProductBaseCode=SL
  Subtract : Subsystem
  phase center reference offset : Constant  Value=fix(mp.maxDelay/2)  OutDataTypeStr=fixdt(0,delayDataTypeWordLength - delayDataTypeFractionLength,0)  SampleTime=-1
  read_addr : Outport  VectorParamsAs1DForOutWhenUnconnected=off
  wires:
  delay/1 -> Subtract/1(In1)
  write_addr/1 -> Subtract/2(In2)
  Increment Real World/1 -> Subtract/3(In3)
  Subtract/1(Out1) -> read_addr/1
  phase center reference offset/1 -> Increment Real World/1

== system gm_DSBF/dataplane/Avalon Data Processing/delay signals_instance10/delay signal/read address generator1 ==
  note: wrap on overflow is the desired behavior
  note: To accommodate positive and negative delays, the read pointer needs to lag the write pointer by the maximum delay + 1. For the maximum positive delay, this puts the read pointer 1 behind the write pointer.
  note: this offset is the maximum possible delay from a microphone to the the center of the array
  write_addr : Inport  OutDataTypeStr=fixdt(0, 6, 0)  PortDimensions=1  SampleTime=1.30208333333333e-06
  delay : Inport  Port=2  OutDataTypeStr=fixdt(1, 6, 0)  PortDimensions=1  SampleTime=1.30208333333333e-06
  Increment Real World : simulink/Additional Math & Discrete/Additional Math: Increment - Decrement/Increment Real World
      settings: SourceProductName=Simulink  SourceProductBaseCode=SL
  Subtract : Subsystem
  phase center reference offset : Constant  Value=fix(mp.upsampleFactor)  OutDataTypeStr=fixdt(0, delayDataTypeFractionLength, 0)  SampleTime=-1
  read_addr : Outport  VectorParamsAs1DForOutWhenUnconnected=off
  wires:
  delay/1 -> Subtract/1(In1)
  write_addr/1 -> Subtract/2(In2)
  Increment Real World/1 -> Subtract/3(In3)
  Subtract/1(Out1) -> read_addr/1
  phase center reference offset/1 -> Increment Real World/1

== system gm_DSBF/dataplane/Avalon Data Processing/delay signals_instance10/delay signal/split_into_int_and_frac_parts ==
  delay : Inport  OutDataTypeStr=fixdt(1, 12, 6)  PortDimensions=1  SampleTime=2.08333333333333e-05
  split_into_int_and_frac_parts : MATLAB Function  TreatAsAtomicUnit=on
  integer_delay : Outport  VectorParamsAs1DForOutWhenUnconnected=off
  fractional_delay : Outport  Port=2
  wires:
  delay/1 -> split_into_int_and_frac_parts/1(delay)
  split_into_int_and_frac_parts/2(fractional_delay) -> fractional_delay/1
  split_into_int_and_frac_parts/1(integer_delay) -> integer_delay/1

== system gm_DSBF/dataplane/Avalon Data Processing/delay signals_instance11/delay signal/read address generator ==
  note: To accommodate positive and negative delays, the read pointer needs to lag the write pointer by the maximum delay + 1. For the maximum positive delay, this puts the read pointer 1 behind the write pointer.
  note: this offset is the maximum possible delay from a microphone to the the center of the array
  note: wrap on overflow is the desired behavior
  write_addr : Inport  OutDataTypeStr=fixdt(0, 6, 0)  PortDimensions=1  SampleTime=2.08333333333333e-05
  delay : Inport  Port=2  OutDataTypeStr=fixdt(1, 6, 0)  PortDimensions=1  SampleTime=2.08333333333333e-05
  Increment Real World : simulink/Additional Math & Discrete/Additional Math: Increment - Decrement/Increment Real World
      settings: SourceProductName=Simulink  SourceProductBaseCode=SL
  Subtract : Subsystem
  phase center reference offset : Constant  Value=fix(mp.maxDelay/2)  OutDataTypeStr=fixdt(0,delayDataTypeWordLength - delayDataTypeFractionLength,0)  SampleTime=-1
  read_addr : Outport  VectorParamsAs1DForOutWhenUnconnected=off
  wires:
  delay/1 -> Subtract/1(In1)
  write_addr/1 -> Subtract/2(In2)
  Increment Real World/1 -> Subtract/3(In3)
  Subtract/1(Out1) -> read_addr/1
  phase center reference offset/1 -> Increment Real World/1

== system gm_DSBF/dataplane/Avalon Data Processing/delay signals_instance11/delay signal/read address generator1 ==
  note: wrap on overflow is the desired behavior
  note: To accommodate positive and negative delays, the read pointer needs to lag the write pointer by the maximum delay + 1. For the maximum positive delay, this puts the read pointer 1 behind the write pointer.
  note: this offset is the maximum possible delay from a microphone to the the center of the array
  write_addr : Inport  OutDataTypeStr=fixdt(0, 6, 0)  PortDimensions=1  SampleTime=1.30208333333333e-06
  delay : Inport  Port=2  OutDataTypeStr=fixdt(1, 6, 0)  PortDimensions=1  SampleTime=1.30208333333333e-06
  Increment Real World : simulink/Additional Math & Discrete/Additional Math: Increment - Decrement/Increment Real World
      settings: SourceProductName=Simulink  SourceProductBaseCode=SL
  Subtract : Subsystem
  phase center reference offset : Constant  Value=fix(mp.upsampleFactor)  OutDataTypeStr=fixdt(0, delayDataTypeFractionLength, 0)  SampleTime=-1
  read_addr : Outport  VectorParamsAs1DForOutWhenUnconnected=off
  wires:
  delay/1 -> Subtract/1(In1)
  write_addr/1 -> Subtract/2(In2)
  Increment Real World/1 -> Subtract/3(In3)
  Subtract/1(Out1) -> read_addr/1
  phase center reference offset/1 -> Increment Real World/1

== system gm_DSBF/dataplane/Avalon Data Processing/delay signals_instance11/delay signal/split_into_int_and_frac_parts ==
  delay : Inport  OutDataTypeStr=fixdt(1, 12, 6)  PortDimensions=1  SampleTime=2.08333333333333e-05
  split_into_int_and_frac_parts : MATLAB Function  TreatAsAtomicUnit=on
  integer_delay : Outport  VectorParamsAs1DForOutWhenUnconnected=off
  fractional_delay : Outport  Port=2
  wires:
  delay/1 -> split_into_int_and_frac_parts/1(delay)
  split_into_int_and_frac_parts/2(fractional_delay) -> fractional_delay/1
  split_into_int_and_frac_parts/1(integer_delay) -> integer_delay/1
